simulink model "zynqRadioWLAN80211BeaconRxAD9361AD9364SL"  (R2016a)
settings: Solver=FixedStepDiscrete  SolverMode=SingleTasking  StartTime=0.0  StopTime=Inf  RelTol=1e-3
PreLoadFcn:
  | load('commwlan80211BusTypes')
  | zynqRadioWLAN80211BeaconRxAD9361AD9364SL_init('init');
  | openMPDUGUI = true;
PostLoadFcn:
  | zynqRadioWLAN80211BeaconRxAD9361AD9364SL_init('scope');
InitFcn:
  | load('commwlan80211BusTypes')
model workspace: external: MAT-File (data not in the file)
undefined symbols (not defined in the file or in its folder): F, gcbh, p80211, rcfiltgaincompat
libraries: commwlan80211BeaconLib x6, sdrzblksprivate x1, commdigbbndpm3 x1, commsequence2 x1, commrfcorlib x1, commfilt2 x1, zc706fmc234_lib x1
CloseFcn:
  | clear BeaconFrameBodyType BeaconMPDUType CapabilityType FrameCtrlType InfoElementType MPDUHeaderType p80211 commwlan80211TxFilt rcvd openMPDUGUI mpduFigPos
  | hFig = findall(0, 'Type', 'figure', 'Name', '802.11 Beacon Frame');
  | if ishghandle(hFig)
  | close(hFig);
  | end
  | clear hFig
  | if (exist('ans')==1) && (iscell(ans) && (numel(ans) == 0))
  | clear ans
  | end
Description:
  | IEEE 802.11b WLAN Beacon Frame Receiver for SDR Hardware
  | 
  | This example shows how to process a beacon frame captured with SDR hardware and display the
  | frame information.
settings Model: ModifiedByFormat=The MathWorks Inc.  SimulationMode=accelerator  Creator=The MathWorks, Inc.  LastModifiedBy=The MathWorks Inc.
settings DataIOCC: LimitDataPoints=on  SaveFormat=Array  SaveOutput=off  SignalLogging=off  DSMLogging=off  SaveTime=off
settings OptimizationCC: DefaultParameterBehavior=Inlined  InlineInvariantSignals=on  ExpressionDepthLimit=2147483647  EfficientFloat2IntCast=on
settings DebuggingCC: UnderspecifiedInitializationDetection=Classic  MergeDetectMultiDrivingBlocksExec=none  SolverPrmCheckMsg=warning  UniqueDataStoreMsg=error  AllowSymbolicDim=off  StateNameClashWarn=warning
settings HardwareCC: ProdBitPerPointer=32  ProdLargestAtomicFloat=None  ProdIntDivRoundTo=Undefined  ProdEndianess=Unspecified  ProdWordSize=32  ProdHWDeviceType=32-bit Generic
settings ModelReferenceCC: PropagateSignalLabelsOutOfModel=off
settings GRTTargetCC: CombineOutputUpdateFcns=off  GRTInterface=on
settings ConfigComp: CovModelRefEnable=Off  CovSFcnEnable=off

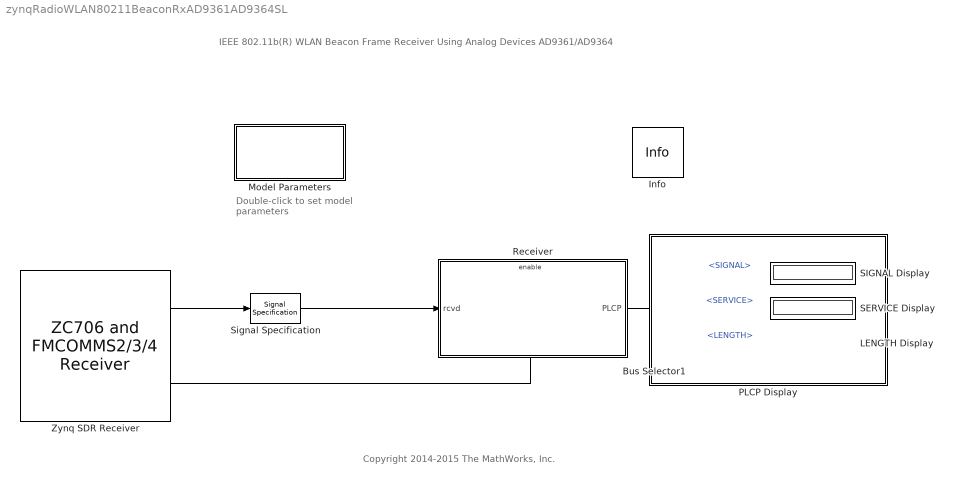
== system zynqRadioWLAN80211BeaconRxAD9361AD9364SL ==
  note: IEEE 802.11b(R) WLAN
      | Beacon Frame Receiver Using Analog Devices AD9361/AD9364
  note: Copyright 2014-2015 The MathWorks, Inc.
  note: Double-click to
      | set model parameters
  Bus Selector1 : BusSelector  OutputSignals=SIGNAL,SERVICE,LENGTH
  Info : sdrzblksprivate/Info  SystemSampleTime=-1
  LENGTH Display : Display
  Model Parameters : Subsystem  mask(Model Parameters){chanNum=11, agcLoopGain=0.0005, agcMaxGain=15, corrThreshold=150, rfGain=20, rfFreqOffset=0, rxFrontendGain=20}
      mask prompts: chanNum "Channel number"; agcLoopGain "AGC loop gain:"; agcMaxGain "Maximum AGC gain:"; corrThreshold "Synchronization threshold:"; rfGain "RF board gain:"; rfFreqOffset "RF center frequency offset:"; rxFrontendGain "Receiver frontend gain"
      mask help:
      | Choose 802.11 receiver parameters.
      |
      | You can select channel number for the 802.11 signals. You can set the AGC parameters and samples per chip used in the receiver. You can also set the synchronization threshold value to determine the correlation threshold used to declare the presence of an 802.11 packet.
      mask init:
      | zynqRadioWLAN80211BeaconRxAD9361AD9364SL_init('init', ...
      |     'ChannelNumber',   chanNum, ...
      |     'AGCLoopGain',     agcLoopGain, ...
      |     'AGCMaxGain',      agcMaxGain, ...
      |     'CorrThreshold',   corrThreshold, ...
      |     'RadioGain',       rfGain, ...
      |     'RadioFreqOffset', rfFreqOffset, ...
      |     'RxFrontendGain',  rxFrontendGain ...
      |     );
      mask TypeOptions chanNum: 1 | 2 | 3 | 4 | 5 | 6 | 7 | 8 | 9 | 10 | 11
      mask Display: disp('Model\nParameters')
  PLCP Display : Subsystem
      mask Display: disp('')
  Receiver : Subsystem
  SERVICE Display : Display
      settings: Format=hex (Stored Integer)
  SIGNAL Display : Display
      settings: Format=hex (Stored Integer)
  Signal Specification : SignalSpecification  SampleTime=p80211.RadioFrameLength/p80211.RadioBasebandRate
  Zynq SDR Receiver : zc706fmc234_lib/ZC706 and  FMCOMMS2//3//4  Receiver  IPAddress=192.168.3.2  CenterFrequencySource=Dialog  CenterFrequency=2.412e9+(p80211.ChannelNumber-1)*5e6+p80211.RadioFreqOffset  GainSource=Dialog  Gain=30  ChannelMapping=1  BasebandSampleRate=p80211.RadioBasebandRate  EnableBurstMode=on  NumFramesInBurst=p80211.RadioNumFramesInBurst  OutputDataType=double  SamplesPerFrame=p80211.RadioFrameLength  LostSamplesOutputPort=off  RSSIOutputPort=off  DMATimeoutValue=1  blockMode=Normal  EnableQuadratureTracking=on  EnableRFDCTracking=on  EnableBasebandDCTracking=on  BypassUserLogic=on  ShowAdvancedProperties=on  ShowInternalProperties=off  subDeviceList=zynqReceiver  sdrExecutionMode=HW  dataUDPPort=-1  ctrlUDPPort=-1  SourceSelect=RF data  SourceConfiguration1=1023  FIRCoefficientSize=[ 128; 128 ]  FIRCoefficients=[ 111, -87, 147, -127, -18, -286, -312, -555, -601, -722, -642, -555, -303, -66, 221, 393, 488, 403, 219, -74, -343, -550, -582, -450, -146, 221, 569, 759, 735, 463, 20, -487, -885, -1048, -883, -418, 243, 897, 1340, 1394, 1002, 228, -715, -1549, -1980, -1819, -1028, 217, 1583, 2635, 2980, 2377, 853, -1275, -3435, -4926, -5080, -3454, 40, 5065, 10903, 16581, 21085, 23573, 23573, 21085, 16581, 10903, 5065, 40, -3454, -5080, -4926, -3435, -1275, 853, 2377, 2980, 2635, 1583, 217, -1028, -1819, -1980, -1549, -715, 228, 1002, 1394, 1340, 897, 243, -418, -883, -1048, -885, -487, 20, 463, 735, 759, 569, 221, -146, -450, -582, -550, -343, -74, 219, 403, 488, 393, 221, -66, -303, -555, -642, -722, -601, -555, -312, -286, -18, -127, 147, -87, 111; 382, -200, 711, -41, 645, 36, 346, -194, -119, -543, -472, -646, -404, -312, 45, 197, 413, 346, 241, -93, -373, -680, -755, -689, -356, 51, 515, 795, 870, 609, 136, -488, -1009, -1303, -1191, -712, 69, 885, 1516, 1692, 1336, 468, -662, -1740, -2378, -2329, -1494, -55, 1620, 2995, 3584, 3045, 1368, -1121, -3755, -5708, -6156, -4542, -710, 4969, 11669, 18243, 23486, 26391, 26391, 23486, 18243, 11669, 4969, -710, -4542, -6156, -5708, -3755, -1121, 1368, 3045, 3584, 2995, 1620, -55, -1494, -2329, -2378, -1740, -662, 468, 1336, 1692, 1516, 885, 69, -712, -1191, -1303, -1009, -488, 136, 609, 870, 795, 515, 51, -356, -689, -755, -680, -373, -93, 241, 346, 413, 197, 45, -312, -404, -646, -472, -543, -119, -194, 346, 36, 645, -41, 711, -200, 382 ]  FIRGain=[ 0; -12 ]  FIRDecimInterpFactor=[ 4; 4 ]  AnalogFilterCutoff=[ 2560000; 2560000 ]  FilterPathRates=[ 737280000, 184320000, 61440000, 30720000, 15360000, 3840000; 737280000, 184320000, 61440000, 30720000, 15360000, 3840000 ]  FilterDesignTypeForTx=DefaultFilterFromOther  FilterDesignTypeForRx=DefaultFilter  BISTLoopbackConfig=No Loopback  BISTPRBSMode=PRBS Disable  BISTToneMode=Tone Disable  BISTToneFrequency=F/32  BISTToneLevel=-6  BISTChannelMask=0  DataIsComplex=on  SimulateUsing=Code generation
  wires:
  Bus Selector1/3 -> LENGTH Display/1  "<LENGTH>"
  Bus Selector1/1 -> SIGNAL Display/1  "<SIGNAL>"
  Bus Selector1/2 -> SERVICE Display/1  "<SERVICE>"
  Receiver/1(PLCP) -> Bus Selector1/1
  Zynq SDR Receiver/2 -> Receiver/Enable
  Zynq SDR Receiver/1 -> Signal Specification/1
  Signal Specification/1 -> Receiver/1(rcvd)

== system zynqRadioWLAN80211BeaconRxAD9361AD9364SL/Model Parameters ==

== system zynqRadioWLAN80211BeaconRxAD9361AD9364SL/PLCP Display ==

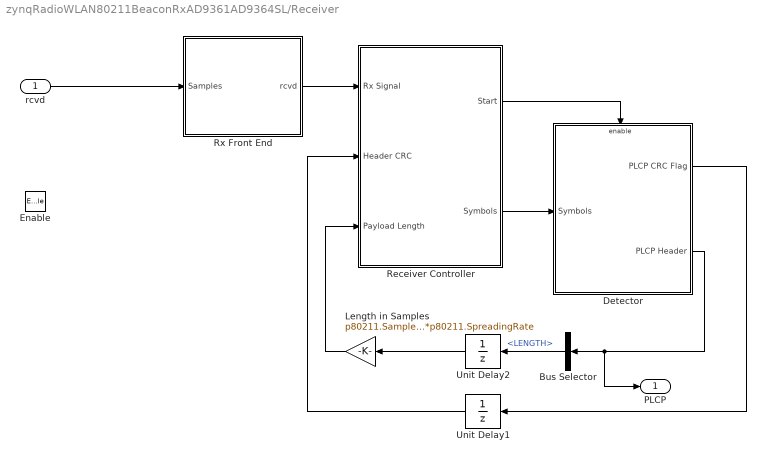
== system zynqRadioWLAN80211BeaconRxAD9361AD9364SL/Receiver ==
  rcvd : Inport
  Enable : EnablePort
  Bus Selector : BusSelector  OutputSignals=LENGTH
  Detector : Subsystem
      settings: CloseFcn=clear BeaconFrameBodyType rcvd
  Length in Samples : Gain  Gain=p80211.SamplesPerChip*p80211.SpreadingRate  OutDataTypeStr=uint32  SaturateOnIntegerOverflow=on  ParamDataTypeStr=Inherit: Same as input
  Receiver Controller : Subsystem
  Rx Front End : Subsystem
  Unit Delay1 : UnitDelay  InitialCondition=1  SampleTime=-1
  Unit Delay2 : UnitDelay  InitialCondition=1  SampleTime=-1
  PLCP : Outport
  wires:
  Receiver Controller/2(Symbols) -> Detector/1(Symbols)
  Detector/2(PLCP Header) -> PLCP/1, Bus Selector/1
  Length in Samples/1 -> Receiver Controller/3(Payload Length)
  Unit Delay2/1 -> Length in Samples/1
  Bus Selector/1 -> Unit Delay2/1  "<LENGTH>"
  Unit Delay1/1 -> Receiver Controller/2(Header CRC)
  Rx Front End/1(rcvd) -> Receiver Controller/1(Rx Signal)
  Detector/1(PLCP CRC Flag) -> Unit Delay1/1
  Receiver Controller/1(Start) -> Detector/Enable
  rcvd/1 -> Rx Front End/1(Samples)

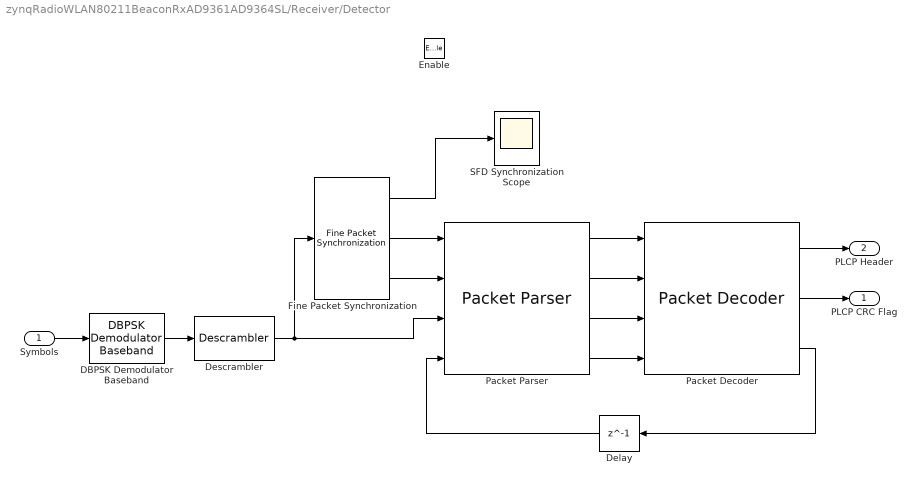
== system zynqRadioWLAN80211BeaconRxAD9361AD9364SL/Receiver/Detector ==
  Symbols : Inport
  Enable : EnablePort  StatesWhenEnabling=reset  PropagateVarSize=During execution
  DBPSK Demodulator Baseband : commdigbbndpm3/DBPSK Demodulator Baseband  Ph=0  outDtype=Smallest unsigned integer
  Delay : Delay  DelayLength=1  InitialCondition=0  InputProcessing=Columns as channels (frame based)
  Descrambler : commsequence2/Descrambler  M=2  poly=p80211.ScramblerPolynomial  iniStaSource=Dialog Parameter  ini_sta=[0 0 0 0 0 0 0]  resetViaPort=off
  Fine Packet Synchronization : commwlan80211BeaconLib/Fine Packet Synchronization
  Packet Decoder : commwlan80211BeaconLib/Packet Decoder
  Packet Parser : commwlan80211BeaconLib/Packet Parser
  SFD Synchronization Scope : Scope
      settings: Priority=10
  PLCP CRC Flag : Outport  InitialOutput=1
  PLCP Header : Outport  Port=2
  wires:
  Packet Decoder/3 -> Delay/1
  Packet Decoder/2 -> PLCP CRC Flag/1
  Packet Decoder/1 -> PLCP Header/1
  Packet Parser/4 -> Packet Decoder/4
  Packet Parser/3 -> Packet Decoder/3
  Packet Parser/2 -> Packet Decoder/2
  Packet Parser/1 -> Packet Decoder/1
  Delay/1 -> Packet Parser/4
  Fine Packet Synchronization/3 -> Packet Parser/2
  Fine Packet Synchronization/2 -> Packet Parser/1
  Descrambler/1 -> Packet Parser/3, Fine Packet Synchronization/1
  Symbols/1 -> DBPSK Demodulator Baseband/1
  DBPSK Demodulator Baseband/1 -> Descrambler/1
  Fine Packet Synchronization/1 -> SFD Synchronization Scope/1

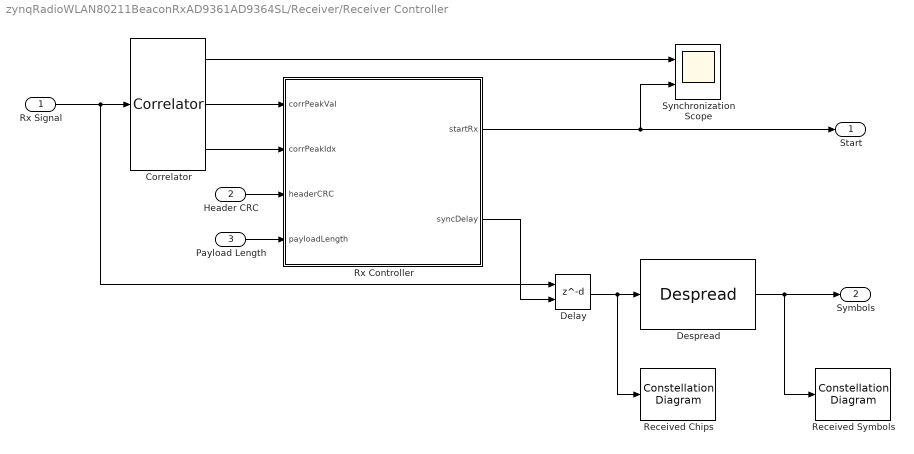
== system zynqRadioWLAN80211BeaconRxAD9361AD9364SL/Receiver/Receiver Controller ==
  Rx Signal : Inport
  Header CRC : Inport  Port=2
  Payload Length : Inport  Port=3
  Correlator : commwlan80211BeaconLib/Correlator
  Delay : Delay  DelayLengthSource=Input port  DelayLengthUpperLimit=p80211.SamplesPerChannelFrame  InputProcessing=Columns as channels (frame based)
      settings: InputPortMap=u0,p1
  Despread : commwlan80211BeaconLib/Despread
  Received Chips : ConstellationDiagram  Tag=ScatterPlot  Priority=1
  Received Symbols : ConstellationDiagram  Tag=ScatterPlot  Priority=2
  Rx Controller : MATLAB Function  TreatAsAtomicUnit=on
  Synchronization Scope : Scope  NumInputPorts=2
      settings: Priority=1
  Start : Outport
  Symbols : Outport  Port=2
  wires:
  Despread/1 -> Received Symbols/1, Symbols/1
  Rx Controller/2(syncDelay) -> Delay/2
  Rx Controller/1(startRx) -> Synchronization Scope/2, Start/1
  Header CRC/1 -> Rx Controller/3(headerCRC)
  Correlator/2 -> Rx Controller/1(corrPeakVal)
  Correlator/3 -> Rx Controller/2(corrPeakIdx)
  Rx Signal/1 -> Correlator/1, Delay/1
  Payload Length/1 -> Rx Controller/4(payloadLength)
  Delay/1 -> Despread/1, Received Chips/1
  Correlator/1 -> Synchronization Scope/1

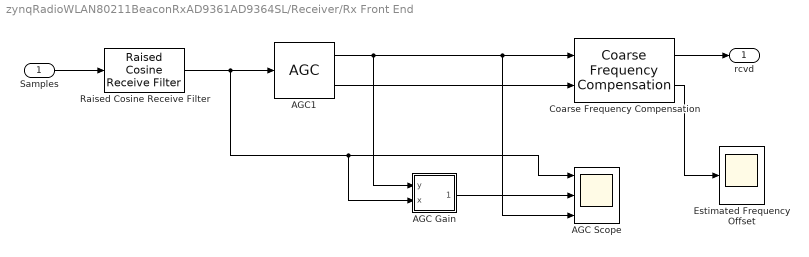
== system zynqRadioWLAN80211BeaconRxAD9361AD9364SL/Receiver/Rx Front End ==
  Samples : Inport
  AGC Gain : Subsystem
  AGC Scope : Scope  NumInputPorts=3
  AGC1 : commrfcorlib/AGC  LegacyMode=off  DetectorMethod=Rectifier  LoopMethod=Linear  UpdatePeriod=100  StepSize=0.1  AdaptationStepSize=p80211.AGCStepSize  DesiredOutputPower=1  AveragingLength=50  MaximumGain=30  MaxPowerGain=p80211.AGCUpperLimit  GainOutputPort=off  InputPowerOutputPort=on  SimulateUsing=Code generation
  Coarse Frequency Compensation : commwlan80211BeaconLib/Coarse Frequency Compensation  decimRate=44  maxOffset=50000  M=2
  Estimated Frequency Offset : Scope
  Raised Cosine Receive Filter : commfilt2/Raised Cosine Receive Filter  filtType=Square root  R=0.3  filtSpan=2*(p80211.FilterOrder/2)  N=p80211.SamplesPerChip  downFactor=1  downOffset=0  filterGain=rcfiltgaincompat(gcbh)  InputProcessing=Columns as channels (frame based)  RateOptions=Enforce single-rate processing  framing=Mute  checkCoeff=off  variableName=rcRxFilt  currentFiltSpan=2*(p80211.FilterOrder/2)  D=p80211.FilterOrder/2  inputOffset=0  sampMode=Mute  saveAsFlag=0  rateMode=Downsampling  checkGain=Normalized  launchFVT=off  roundingMode=Floor  overflowMode=off  coeffDataTypeStr=Inherit: Same word length as input  coeffMin=[]  coeffMax=[]  coeffLastDataTypeStr=Inherit: Same word length as input  accumDataTypeStr=Inherit: Same as product output  accumLastDataTypeStr=Inherit: Same as product output  outputDataTypeStr=Inherit: Same as accumulator  outputMin=[]  outputMax=[]  outputLastDataTypeStr=Inherit: Same as accumulator
  rcvd : Outport
  wires:
  Coarse Frequency Compensation/1 -> rcvd/1
  AGC1/1 -> AGC Gain/1(y), Coarse Frequency Compensation/1, AGC Scope/3
  Raised Cosine Receive Filter/1 -> AGC Gain/2(x), AGC Scope/1, AGC1/1
  Coarse Frequency Compensation/2 -> Estimated Frequency Offset/1
  AGC1/2 -> Coarse Frequency Compensation/2
  Samples/1 -> Raised Cosine Receive Filter/1
  AGC Gain/1(gain) -> AGC Scope/2

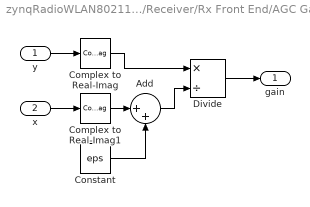
== system zynqRadioWLAN80211BeaconRxAD9361AD9364SL/Receiver/Rx Front End/AGC Gain ==
  y : Inport
  x : Inport  Port=2
  Add : Sum  Inputs=|++
  Complex to Real-Imag : ComplexToRealImag  Output=Real
  Complex to Real-Imag1 : ComplexToRealImag  Output=Real
  Constant : Constant  Value=eps
  Divide : Product  Inputs=*/
  gain : Outport
  wires:
  Divide/1 -> gain/1
  y/1 -> Complex to Real-Imag/1
  x/1 -> Complex to Real-Imag1/1
  Complex to Real-Imag/1 -> Divide/1
  Complex to Real-Imag1/1 -> Add/1
  Add/1 -> Divide/2
  Constant/1 -> Add/2

== matlab function zynqRadioWLAN80211BeaconRxAD9361AD9364SL/Receiver/Receiver Controller/Rx Controller ==
  data: corrPeakVal input; startRx output; corrPeakIdx input; headerCRC input boolean size=[1 1]; payloadLength input size=1; p80211 parameter; syncDelay output
function [startRx, syncDelay] = ...
  rxCtrl(corrPeakVal, corrPeakIdx, headerCRC, payloadLength, p80211)
%#codegen

persistent rxOn controllerState payloadCount lastSyncDelay corrPeakValOld

% State Enums
SearchPLCP = 0;
GetPLCP    = 2;
GetPayload = 4;

if isempty(rxOn)
  % Initialize receiver controller
  rxOn = false;
  controllerState = SearchPLCP;
  payloadCount = 0;
  lastSyncDelay = 0;
  corrPeakValOld = 0;
end

if (corrPeakValOld < corrPeakVal)
  controllerState = SearchPLCP;
end

switch controllerState
  case SearchPLCP
    % Search for the PLCP SYNC signal
    
    if corrPeakVal > p80211.CorrelationThreshold
      corrPeakValOld = corrPeakVal;
      % Synchronize to the end of the SYNC. Get 8 (scrambler length) extra
      % bits to initialize DPSK demodulator and scrambler
      scramblerLen = length(p80211.ScramblerPolynomial);
      lastSyncDelay = p80211.SamplesPerChannelFrame - (corrPeakIdx ...
        - scramblerLen*p80211.SpreadingRate*p80211.SamplesPerChip); 
      payloadCount = p80211.NumSYNCSamples ...
        - scramblerLen*p80211.SpreadingRate*p80211.SamplesPerChip;
      rxOn = true;
      
      controllerState = GetPLCP;
    end
  case GetPLCP
    % In this state we receive both SFD, which is part of PLCP preamble,
    % and the PLCP header
    
    payloadCount = payloadCount + p80211.SamplesPerChannelFrame;
    
    if (payloadCount >= ...
        (p80211.NumPLCPSamples+p80211.ScramblerAmbiguitySamples))
      if headerCRC ~= 1
        controllerState = GetPayload;
      else
        rxOn = false;
        lastSyncDelay = 0;
        payloadCount = 0;
        controllerState = SearchPLCP;
      end
    end
  case GetPayload
    % Receive payload symbols
    
    payloadCount = payloadCount + p80211.SamplesPerChannelFrame;
    
    if payloadCount >= ...
        ((p80211.NumPLCPSamples+p80211.ScramblerAmbiguitySamples) + ...
        payloadLength)
      rxOn = false;
      lastSyncDelay = 0;
      payloadCount = 0;
      controllerState = SearchPLCP;
    end
end

startRx = rxOn;
syncDelay = lastSyncDelay;
